simulink model "Kite_sim_actuation"  (R2022b)
settings: Solver=ode15s  StartTime=0.0  StopTime=120  FixedStep=Ts_10ms  RelTol=1e-3
InitFcn:
  | clc
  | eval('SimPrm')
StopFcn:
  | figure,plot3(Position.signals.values(:,1),Position.signals.values(:,2),Position.signals.values(:,3),'k'),grid on,hold on
  | plot3(0,0,0,'k*')
  | plot3([0, Position.signals.values(end,1)],...
  |       [0, Position.signals.values(end,2)],...
  |       [0, Position.signals.values(end,3)], 'b-o')
  | xlabel('X (m)'), ylabel('Y (m)'), zlabel('Z (m)')
  | SmoothWindPlot
values from neighbouring files (symbols this model uses):
  alpha_0 = 2.5*pi/180    (= 0.0436332312999)    [SimPrm.m]
  alpha_max = 18*pi/180    (= 0.314159265359)    [SimPrm.m]
  alpha_min = -8*pi/180    (= -0.13962634016)    [SimPrm.m]
  alpha_var = [-8.5 0 6 10 14 16 18 20]*pi/180'    [SimPrm.m]
  area = 9    [SimPrm.m]
  CD_Line = 1.2    [SimPrm.m]
  CD_var = [0.010 0.013 0.048 0.083     0.128 0.154 0.181 0.218]'    [SimPrm.m]
  CL_var = [-0.147 0.332 0.652 0.838     0.99 1.052 1.084 1.032]'*0.8    [SimPrm.m]
  ConstWindX = 5    [SimPrm.m]
  ConstWindY = 0    [SimPrm.m]
  ConstWindZ = 0    [SimPrm.m]
  g = 9.81    [SimPrm.m]
  gamma_fb_K = 2*2.8*0.01    (= 0.056)    [SimPrm.m]
  HLC2dl = -4    [SimPrm.m]
  HLC_input_max = 0.25    [SimPrm.m]
  init_stat = [60*pi/180 1*pi/180      1*pi/180 1*pi/180      50 0]    [SimPrm.m]
  K_r = 1000    [SimPrm.m]
  Line_density = 970    [SimPrm.m]
  Line_diameter = 0.003    [SimPrm.m]
  mass = 2.4    [SimPrm.m]
  n_line = 3    [SimPrm.m]
  r_ref = init_stat(5)    [SimPrm.m]
  rho = 1.2    [SimPrm.m]
  Targets_matrix = [0.3 -0.3 ... (first row only)    [SimPrm.m]
  Ts_10ms = 1e-2    (= 0.01)    [SimPrm.m]
  wingspan = 2    [SimPrm.m]
undefined symbols (not defined in the file or in its folder): WxFncH, WyFncH
settings Model: PauseTimes=60  Creator=Philip Hu  LastModifiedBy=matte
settings SolverCC: AlgebraicLoopSolver=TrustRegion  MinimalZcImpactIntegration=on
settings DataIOCC: SaveFormat=Array  SignalLoggingSaveFormat=ModelDataLogs  SaveOutput=off  SignalLogging=off  SaveTime=off  ReturnWorkspaceOutputs=off
settings OptimizationCC: BufferReuse=off  GlobalBufferReuse=off  ExpressionFolding=off  ExpressionDepthLimit=2147483647  LocalBlockOutputs=off
settings DebuggingCC: ReadBeforeWriteMsg=DisableAll  WriteAfterWriteMsg=DisableAll  WriteAfterReadMsg=DisableAll  UnderspecifiedInitializationDetection=Classic  MergeDetectMultiDrivingBlocksExec=none  SolverPrmCheckMsg=warning  MultiTaskDSMMsg=none  UnconnectedInputMsg=warning  UnconnectedOutputMsg=warning  UnconnectedLineMsg=warning  StateNameClashWarn=warning  SFUnexpectedBacktrackingDiag=warning  SFNoUnconditionalDefaultTransitionDiag=warning  SFExecutionAtInitializationDiag=none  ArithmeticOperatorsInVariantConditions=warning
settings HardwareCC: ProdBitPerPointer=32  ProdBitPerSizeT=32  ProdBitPerPtrDiffT=32  ProdLargestAtomicFloat=None  ProdWordSize=32  ProdLongLongMode=on  ProdHWDeviceType=Generic->32-bit x86 compatible
settings ModelReferenceCC: UpdateModelReferenceTargets=IfOutOfDate  EnableRefExpFcnMdlSchedulingChecks=on  PropagateSignalLabelsOutOfModel=off
settings SFSimCC: SFSimEcho=off  SimUseLocalCustomCode=off  SimParseCustomCode=off  CustomCodeUndefinedFunction=UseInterfaceOnly
settings RTWCC: Description=Simulink Real-Time  SystemTargetFile=slrt.tlc  TemplateMakefile=slrt_default_tmf  RTWUseLocalCustomCode=off  RTWCompilerOptimization=on
settings CodeAppCC: StateflowObjectComments=on
settings SimulinkRealTimeCC: OptimizeReductions=off  RL32ObjectName=HAWE  xPCisModelTimeout=off  xPCModelTimeoutSecs=20
settings ConfigComp: CovMetricSettings=dw  CovSaveCumulativeToWorkspaceVar=on  CovSaveSingleToWorkspaceVar=on  CovExternalEMLEnable=off

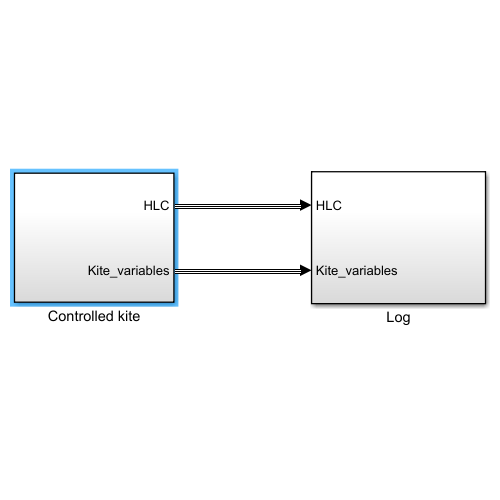
[thumbnail: Simulink's stored preview of the top-level diagram]
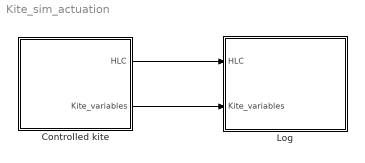
== system Kite_sim_actuation ==
  Controlled kite : Subsystem
  Log : Subsystem
  wires:
  Controlled kite/1(HLC) -> Log/1(HLC)
  Controlled kite/2(Kite_variables) -> Log/2(Kite_variables)

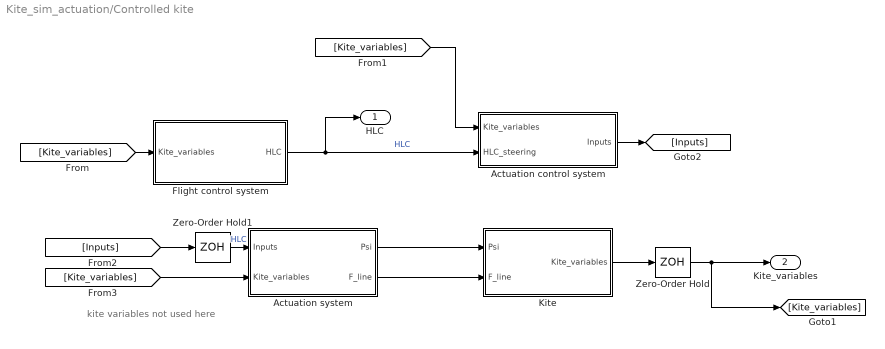
== system Kite_sim_actuation/Controlled kite ==
  note: kite variables not used here
  Actuation control system : Subsystem
  Actuation system : Subsystem
  Flight control system : Subsystem
  Kite : Subsystem
  Zero-Order Hold : ZeroOrderHold  SampleTime=Ts_10ms
  Zero-Order Hold1 : ZeroOrderHold  SampleTime=Ts_10ms
  HLC : Outport
  Kite_variables : Outport  Port=2
  wires:
  Kite/1(Kite_variables) -> Zero-Order Hold/1
  Flight control system/1(HLC) -> Actuation control system/2(HLC_steering), HLC/1  "HLC"
  Zero-Order Hold/1 -> [Kite_variables], Kite_variables/1
  [Kite_variables] -> Flight control system/1(Kite_variables)
  [Kite_variables] -> Actuation control system/1(Kite_variables)
  Actuation control system/1(Inputs) -> [Inputs]
  [Inputs] -> Zero-Order Hold1/1
  Zero-Order Hold1/1 -> Actuation system/1(Inputs)  "HLC"
  Actuation system/2(F_line) -> Kite/2(F_line)
  Actuation system/1(Psi) -> Kite/1(Psi)
  [Kite_variables] -> Actuation system/2(Kite_variables)

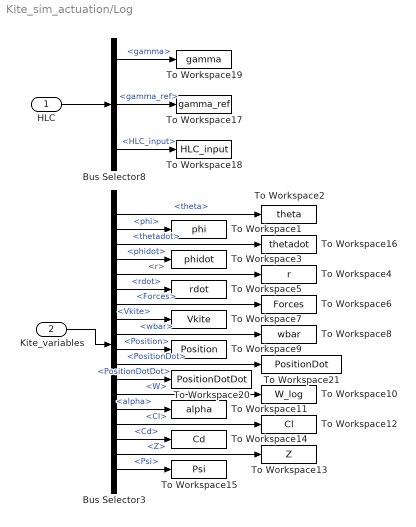
== system Kite_sim_actuation/Log ==
  HLC : Inport
  Kite_variables : Inport  Port=2
  Bus Selector3 : BusSelector  OutputSignals=states.theta,states.phi,states.thetadot,states.phidot,states.r,states.rdot,Forces,Vkite,wbar,Position,PositionDot,PositionDotDot,W,alpha,Cl,Cd,Z,Psi
  Bus Selector8 : BusSelector  OutputSignals=gamma,gamma_ref,HLC_input
  To Workspace1 : ToWorkspace  VariableName=phi  SaveFormat=Structure With Time  SampleTime=-1
  To Workspace10 : ToWorkspace  VariableName=W_log  SaveFormat=Structure With Time  SampleTime=-1
  To Workspace11 : ToWorkspace  VariableName=alpha  SaveFormat=Structure With Time  SampleTime=-1
  To Workspace12 : ToWorkspace  VariableName=Cl  SaveFormat=Structure With Time  SampleTime=-1
  To Workspace13 : ToWorkspace  VariableName=Z  SaveFormat=Structure With Time  SampleTime=-1
  To Workspace14 : ToWorkspace  VariableName=Cd  SaveFormat=Structure With Time  SampleTime=-1
  To Workspace15 : ToWorkspace  VariableName=Psi  SaveFormat=Structure With Time  SampleTime=-1
  To Workspace16 : ToWorkspace  VariableName=thetadot  SaveFormat=Structure With Time  SampleTime=-1
  To Workspace17 : ToWorkspace  VariableName=gamma_ref  SaveFormat=Structure With Time  SampleTime=-1
  To Workspace18 : ToWorkspace  VariableName=HLC_input  SaveFormat=Structure With Time  SampleTime=-1
  To Workspace19 : ToWorkspace  VariableName=gamma  SaveFormat=Structure With Time  SampleTime=-1
  To Workspace2 : ToWorkspace  VariableName=theta  SaveFormat=Structure With Time  SampleTime=-1
  To Workspace20 : ToWorkspace  VariableName=PositionDotDot  SaveFormat=Structure With Time  SampleTime=-1
  To Workspace21 : ToWorkspace  VariableName=PositionDot  SaveFormat=Structure With Time  SampleTime=-1
  To Workspace3 : ToWorkspace  VariableName=phidot  SaveFormat=Structure With Time  SampleTime=-1
  To Workspace4 : ToWorkspace  VariableName=r  SaveFormat=Structure With Time  SampleTime=-1
  To Workspace5 : ToWorkspace  VariableName=rdot  SaveFormat=Structure With Time  SampleTime=-1
  To Workspace6 : ToWorkspace  VariableName=Forces  SaveFormat=Structure With Time  SampleTime=-1
  To Workspace7 : ToWorkspace  VariableName=Vkite  SaveFormat=Structure With Time  SampleTime=-1
  To Workspace8 : ToWorkspace  VariableName=wbar  SaveFormat=Structure With Time  SampleTime=-1
  To Workspace9 : ToWorkspace  VariableName=Position  SaveFormat=Structure With Time  SampleTime=-1
  wires:
  HLC/1 -> Bus Selector8/1
  Kite_variables/1 -> Bus Selector3/1
  Bus Selector3/5 -> To Workspace4/1  "<r>"
  Bus Selector3/6 -> To Workspace5/1  "<rdot>"
  Bus Selector3/7 -> To Workspace6/1  "<Forces>"
  Bus Selector3/8 -> To Workspace7/1  "<Vkite>"
  Bus Selector3/9 -> To Workspace8/1  "<wbar>"
  Bus Selector3/10 -> To Workspace9/1  "<Position>"
  Bus Selector3/13 -> To Workspace10/1  "<W>"
  Bus Selector3/14 -> To Workspace11/1  "<alpha>"
  Bus Selector3/15 -> To Workspace12/1  "<Cl>"
  Bus Selector3/16 -> To Workspace14/1  "<Cd>"
  Bus Selector3/18 -> To Workspace15/1  "<Psi>"
  Bus Selector3/1 -> To Workspace2/1  "<theta>"
  Bus Selector3/2 -> To Workspace1/1  "<phi>"
  Bus Selector3/4 -> To Workspace3/1  "<phidot>"
  Bus Selector3/17 -> To Workspace13/1  "<Z>"
  Bus Selector3/3 -> To Workspace16/1  "<thetadot>"
  Bus Selector8/3 -> To Workspace18/1  "<HLC_input>"
  Bus Selector8/2 -> To Workspace17/1  "<gamma_ref>"
  Bus Selector8/1 -> To Workspace19/1  "<gamma>"
  Bus Selector3/12 -> To Workspace20/1  "<PositionDotDot>"
  Bus Selector3/11 -> To Workspace21/1  "<PositionDot>"

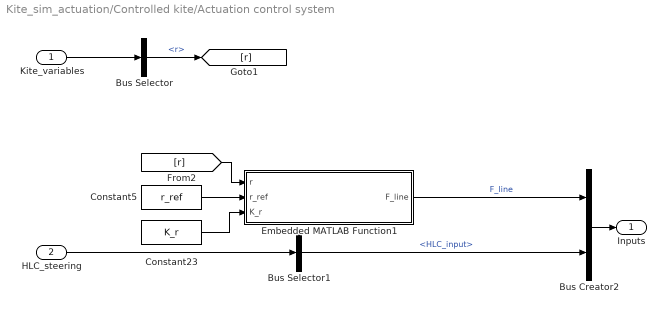
== system Kite_sim_actuation/Controlled kite/Actuation control system ==
  Kite_variables : Inport
  HLC_steering : Inport  Port=2
  Bus Creator2 : BusCreator  Inputs=2
  Bus Selector : BusSelector  OutputSignals=states.r
  Bus Selector1 : BusSelector  OutputSignals=HLC_input
  Constant23 : Constant  Value=K_r
  Constant5 : Constant  Value=r_ref
  Embedded MATLAB Function1 : MATLAB Function  TreatAsAtomicUnit=on
  Inputs : Outport
  wires:
  Embedded MATLAB Function1/1(F_line) -> Bus Creator2/1  "F_line"
  [r] -> Embedded MATLAB Function1/1(r)
  Constant5/1 -> Embedded MATLAB Function1/2(r_ref)
  Constant23/1 -> Embedded MATLAB Function1/3(K_r)
  Kite_variables/1 -> Bus Selector/1
  Bus Selector/1 -> [r]  "<r>"
  HLC_steering/1 -> Bus Selector1/1
  Bus Creator2/1 -> Inputs/1
  Bus Selector1/1 -> Bus Creator2/2  "<HLC_input>"

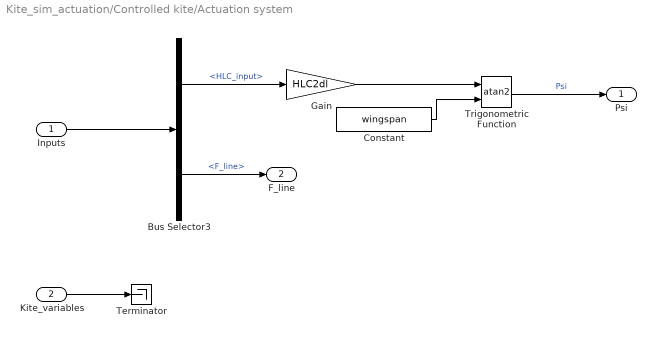
== system Kite_sim_actuation/Controlled kite/Actuation system ==
  Inputs : Inport
  Kite_variables : Inport  Port=2
  Bus Selector3 : BusSelector  OutputSignals=HLC_input,F_line
  Constant : Constant  Value=wingspan
  Gain : Gain  Gain=HLC2dl
  Terminator : Terminator
  Trigonometric Function : Trigonometry  Operator=atan2
  Psi : Outport
  F_line : Outport  Port=2
  wires:
  Bus Selector3/1 -> Gain/1  "<HLC_input>"
  Trigonometric Function/1 -> Psi/1  "Psi"
  Constant/1 -> Trigonometric Function/2
  Gain/1 -> Trigonometric Function/1
  Inputs/1 -> Bus Selector3/1
  Bus Selector3/2 -> F_line/1  "<F_line>"
  Kite_variables/1 -> Terminator/1

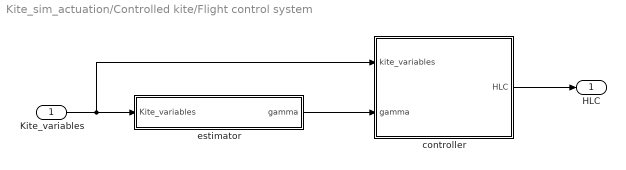
== system Kite_sim_actuation/Controlled kite/Flight control system ==
  Kite_variables : Inport
  controller : Subsystem
  estimator : Subsystem
  HLC : Outport
  wires:
  estimator/1(gamma) -> controller/2(gamma)
  controller/1(HLC) -> HLC/1
  Kite_variables/1 -> estimator/1(Kite_variables), controller/1(kite_variables)

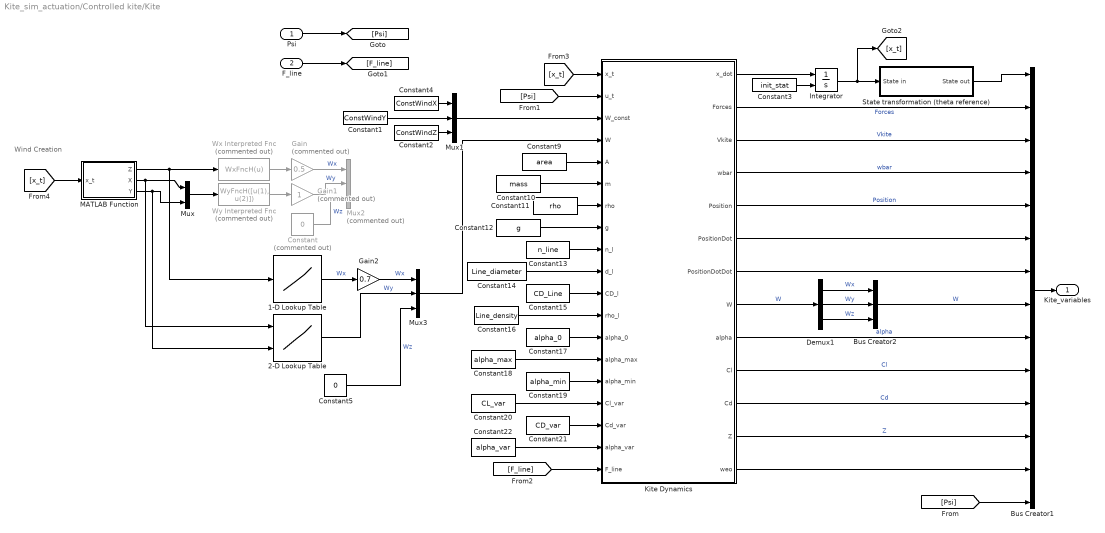
== system Kite_sim_actuation/Controlled kite/Kite ==
  note: Wind Creation
  Psi : Inport
  F_line : Inport  Port=2
  1-D Lookup Table : Lookup_n-D  NumberOfTableDimensions=1  BreakpointsForDimension1=[0;5;10;15;20;25;40;50]  Table=[0 2 8 10 12 20 20 20]  InterpMethod=Cubic spline  ExtrapMethod=Cubic spline  InternalRulePriority=Speed  RndMeth=Simplest
  2-D Lookup Table : Lookup_n-D  BreakpointsForDimension1=[0 25 30 50 60 80 100]  BreakpointsForDimension2=[-50;-20;-10;0;10;20;50]  Table=[0 0 0 0 0 0 0;0 0 0 0 0 0 0;0 0 5 0 0 0 0;0 0 0 0 10 0 0;0 0 0 0 0 0 0;0 -10 0 0 0 0 0;0 0 0 0 0 0 0]  InterpMethod=Cubic spline  ExtrapMethod=Cubic spline  InternalRulePriority=Speed  RndMeth=Simplest
      settings: InputPortMap=u0,u1
  Bus Creator1 : BusCreator  Inputs=14
  Bus Creator2 : BusCreator  Inputs=3
  Constant : Constant  Commented=on  Value=0
  Constant1 : Constant  Value=ConstWindY
  Constant10 : Constant  Value=mass
  Constant11 : Constant  Value=rho
  Constant12 : Constant  Value=g
  Constant13 : Constant  Value=n_line
  Constant14 : Constant  Value=Line_diameter
  Constant15 : Constant  Value=CD_Line
  Constant16 : Constant  Value=Line_density
  Constant17 : Constant  Value=alpha_0
  Constant18 : Constant  Value=alpha_max
  Constant19 : Constant  Value=alpha_min
  Constant2 : Constant  Value=ConstWindZ
  Constant20 : Constant  Value=CL_var
  Constant21 : Constant  Value=CD_var
  Constant22 : Constant  Value=alpha_var
  Constant3 : Constant  Value=init_stat
  Constant4 : Constant  Value=ConstWindX
  Constant5 : Constant  Value=0
  Constant9 : Constant  Value=area
  Demux1 : Demux  Outputs=3
  Gain : Gain  Commented=on  Gain=0.5
  Gain1 : Gain  Commented=on
  Gain2 : Gain  Gain=0.7
  Integrator : Integrator  InitialConditionSource=external
  Kite Dynamics : MATLAB Function  TreatAsAtomicUnit=on
  MATLAB Function : MATLAB Function  TreatAsAtomicUnit=on
  Mux : Mux  Inputs=2
  Mux1 : Mux  Inputs=3
  Mux2 : Mux  Commented=on  Inputs=3
  Mux3 : Mux  Inputs=3
  State transformation (theta reference) : Subsystem
  Wx Interpreted Fnc : MATLABFcn  Commented=on  MATLABFcn=WxFncH(u)  OutputDimensions=1  OutputSignalType=real  Output1D=off
  Wy Interpreted Fnc : MATLABFcn  Commented=on  MATLABFcn=WyFncH([u(1), u(2)])  OutputDimensions=1  OutputSignalType=real  Output1D=off
  Kite_variables : Outport
  wires:
  State transformation (theta reference)/1(State out) -> Bus Creator1/1
  Constant2/1 -> Mux1/3
  Constant1/1 -> Mux1/2
  Constant4/1 -> Mux1/1
  Mux1/1 -> Kite Dynamics/3(W_const)
  Constant9/1 -> Kite Dynamics/5(A)
  Constant10/1 -> Kite Dynamics/6(m)
  Constant11/1 -> Kite Dynamics/7(rho)
  Constant12/1 -> Kite Dynamics/8(g)
  Constant13/1 -> Kite Dynamics/9(n_l)
  Constant14/1 -> Kite Dynamics/10(d_l)
  Constant15/1 -> Kite Dynamics/11(CD_l)
  Constant16/1 -> Kite Dynamics/12(rho_l)
  Constant18/1 -> Kite Dynamics/14(alpha_max)
  Constant20/1 -> Kite Dynamics/16(Cl_var)
  Constant22/1 -> Kite Dynamics/18(alpha_var)
  Constant17/1 -> Kite Dynamics/13(alpha_0)
  Constant19/1 -> Kite Dynamics/15(alpha_min)
  Constant21/1 -> Kite Dynamics/17(Cd_var)
  [F_line] -> Kite Dynamics/19(F_line)
  Bus Creator1/1 -> Kite_variables/1
  Kite Dynamics/2(Forces) -> Bus Creator1/2  "Forces"
  Kite Dynamics/3(Vkite) -> Bus Creator1/3  "Vkite"
  Kite Dynamics/4(wbar) -> Bus Creator1/4  "wbar"
  Kite Dynamics/5(Position) -> Bus Creator1/5  "Position"
  Kite Dynamics/8(W) -> Demux1/1  "W"
  Kite Dynamics/9(alpha) -> Bus Creator1/9  "alpha"
  Kite Dynamics/10(Cl) -> Bus Creator1/10  "Cl"
  Kite Dynamics/11(Cd) -> Bus Creator1/11  "Cd"
  Kite Dynamics/12(Z) -> Bus Creator1/12  "Z"
  Integrator/1 -> [x_t], State transformation (theta reference)/1(State in)
  Constant3/1 -> Integrator/2
  Kite Dynamics/1(x_dot) -> Integrator/1
  Kite Dynamics/13(weo) -> Bus Creator1/13
  Demux1/1 -> Bus Creator2/1  "Wx"
  Demux1/2 -> Bus Creator2/2  "Wy"
  Demux1/3 -> Bus Creator2/3  "Wz"
  Bus Creator2/1 -> Bus Creator1/8  "W"
  [Psi] -> Bus Creator1/14
  [Psi] -> Kite Dynamics/2(u_t)
  Psi/1 -> [Psi]
  F_line/1 -> [F_line]
  Constant/1 -> Mux2/3  "Wz"
  MATLAB Function/1(Z) -> 1-D Lookup Table/1, Wx Interpreted Fnc/1
  Mux/1 -> Wy Interpreted Fnc/1
  MATLAB Function/2(X) -> 2-D Lookup Table/1, Mux/1
  MATLAB Function/3(Y) -> 2-D Lookup Table/2, Mux/2
  Wx Interpreted Fnc/1 -> Gain/1
  Gain/1 -> Mux2/1  "Wx"
  Wy Interpreted Fnc/1 -> Gain1/1
  Gain1/1 -> Mux2/2  "Wy"
  [x_t] -> Kite Dynamics/1(x_t)
  [x_t] -> MATLAB Function/1(x_t)
  2-D Lookup Table/1 -> Mux3/2  "Wy"
  1-D Lookup Table/1 -> Gain2/1  "Wx"
  Constant5/1 -> Mux3/3  "Wz"
  Mux3/1 -> Kite Dynamics/4("W ")
  Gain2/1 -> Mux3/1  "Wx"
  Kite Dynamics/7(PositionDotDot) -> Bus Creator1/7
  Kite Dynamics/6(PositionDot) -> Bus Creator1/6

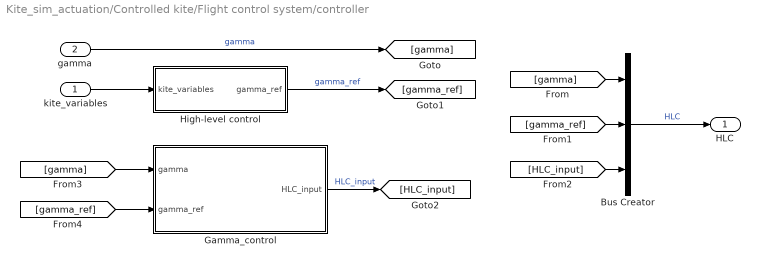
== system Kite_sim_actuation/Controlled kite/Flight control system/controller ==
  kite_variables : Inport
  gamma : Inport  Port=2
  Bus Creator : BusCreator  Inputs=3
  Gamma_control : Subsystem
  High-level control : Subsystem
  HLC : Outport
  wires:
  Bus Creator/1 -> HLC/1  "HLC"
  High-level control/1(gamma_ref) -> [gamma_ref]  "gamma_ref"
  kite_variables/1 -> High-level control/1(kite_variables)
  gamma/1 -> [gamma]  "gamma"
  [gamma] -> Bus Creator/1
  Gamma_control/1(HLC_input) -> [HLC_input]  "HLC_input"
  [gamma_ref] -> Bus Creator/2
  [HLC_input] -> Bus Creator/3
  [gamma] -> Gamma_control/1(gamma)
  [gamma_ref] -> Gamma_control/2(gamma_ref)

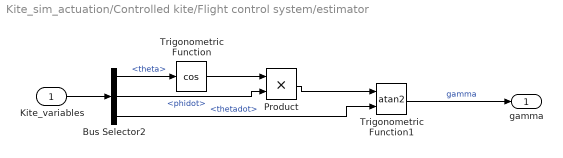
== system Kite_sim_actuation/Controlled kite/Flight control system/estimator ==
  Kite_variables : Inport
  Bus Selector2 : BusSelector  OutputSignals=states.theta,states.phidot,states.thetadot
  Product : Product  RndMeth=Zero
  Trigonometric Function : Trigonometry  Operator=cos
  Trigonometric Function1 : Trigonometry  Operator=atan2
  gamma : Outport
  wires:
  Kite_variables/1 -> Bus Selector2/1
  Bus Selector2/3 -> Trigonometric Function1/2  "<thetadot>"
  Bus Selector2/1 -> Trigonometric Function/1  "<theta>"
  Bus Selector2/2 -> Product/2  "<phidot>"
  Product/1 -> Trigonometric Function1/1
  Trigonometric Function1/1 -> gamma/1  "gamma"
  Trigonometric Function/1 -> Product/1

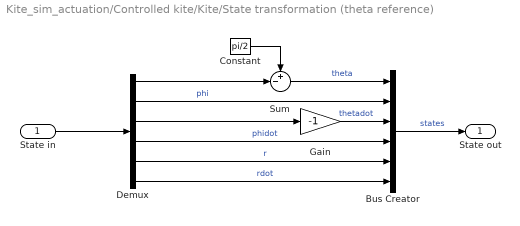
== system Kite_sim_actuation/Controlled kite/Kite/State transformation (theta reference) ==
  State in : Inport
  Bus Creator : BusCreator  Inputs=6
  Constant : Constant  Value=pi/2
  Demux : Demux  Outputs=6
  Gain : Gain  Gain=-1
  Sum : Sum  Inputs=+-|
  State out : Outport
  wires:
  Demux/2 -> Bus Creator/2  "phi"
  Demux/3 -> Gain/1
  Demux/4 -> Bus Creator/4  "phidot"
  Demux/5 -> Bus Creator/5  "r"
  Demux/6 -> Bus Creator/6  "rdot"
  Constant/1 -> Sum/1
  Demux/1 -> Sum/2
  Sum/1 -> Bus Creator/1  "theta"
  Gain/1 -> Bus Creator/3  "thetadot"
  State in/1 -> Demux/1
  Bus Creator/1 -> State out/1  "states"

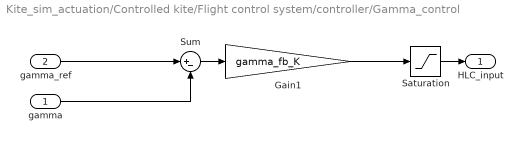
== system Kite_sim_actuation/Controlled kite/Flight control system/controller/Gamma_control ==
  gamma : Inport
  gamma_ref : Inport  Port=2
  Gain1 : Gain  Gain=gamma_fb_K
  Saturation : Saturate  UpperLimit=HLC_input_max  LowerLimit=-HLC_input_max
  Sum : Sum  Inputs=|+-
  HLC_input : Outport
  wires:
  Sum/1 -> Gain1/1
  Gain1/1 -> Saturation/1
  gamma_ref/1 -> Sum/1
  Saturation/1 -> HLC_input/1
  gamma/1 -> Sum/2

== system Kite_sim_actuation/Controlled kite/Flight control system/controller/High-level control ==
  kite_variables : Inport
  Bus Selector3 : BusSelector  OutputSignals=states.theta,states.phi
  Guidance : Subsystem
  gamma_ref : Outport
  wires:
  kite_variables/1 -> Bus Selector3/1
  Bus Selector3/1 -> Guidance/1(theta)  "<theta>"
  Bus Selector3/2 -> Guidance/2(phi)  "<phi>"
  Guidance/1(gamma_ref) -> gamma_ref/1  "gamma_ref"

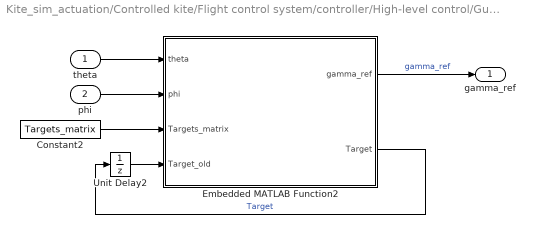
== system Kite_sim_actuation/Controlled kite/Flight control system/controller/High-level control/Guidance ==
  theta : Inport
  phi : Inport  Port=2
  Constant2 : Constant  Value=Targets_matrix
  Embedded MATLAB Function2 : MATLAB Function  TreatAsAtomicUnit=on
  Unit Delay2 : UnitDelay  InitialCondition=1  SampleTime=-1  HasFrameUpgradeWarning=on
  gamma_ref : Outport
  wires:
  Embedded MATLAB Function2/1(gamma_ref) -> gamma_ref/1  "gamma_ref"
  Embedded MATLAB Function2/2(Target) -> Unit Delay2/1  "Target"
  theta/1 -> Embedded MATLAB Function2/1(theta)
  phi/1 -> Embedded MATLAB Function2/2(phi)
  Constant2/1 -> Embedded MATLAB Function2/3(Targets_matrix)
  Unit Delay2/1 -> Embedded MATLAB Function2/4(Target_old)

== matlab function Kite_sim_actuation/Controlled kite/Flight control system/controller/High-level control/Guidance/Embedded MATLAB Function2 ==
  data: theta input; phi input; Targets_matrix input; gamma_ref output; Target output; Target_old input
function [gamma_ref,Target]=kite_guidance(theta,...
                                         phi,...
                                         Targets_matrix,...
                                         Target_old)%#eml

% Gamma reference computation strategy (based on theta, phi and Target; 
% theta and phi of the targets to be included in Targets_matrix, 
% e.g. the i-th row has theta and phi of the 
% i-th target; theta_min is for emergency situation)

if phi > Targets_matrix(2,2) % Regular switch, over pos limit
    Target = 1;
elseif phi < Targets_matrix(1,2) % Regular switch, below neg limit
    Target = 2;
else
    Target = Target_old;
end

% Calculate gamma_ref
theta_t = Targets_matrix(Target,1);
phi_t   = Targets_matrix(Target,2);
gamma_ref = atan2((phi_t - phi)*cos(theta),theta_t - theta);

== matlab function Kite_sim_actuation/Controlled kite/Actuation control system/Embedded MATLAB Function1 ==
  data: r input; F_line output; r_ref input; K_r input
function F_line=...
    line_ctrl(r,r_ref,K_r)%#eml


F_line=[0;0;-K_r*(r_ref-r)];
F_line(3,1)=max(0,F_line(3,1)); % cable traction force (always positive and subtracted to other forces)

== matlab function Kite_sim_actuation/Controlled kite/Kite/MATLAB Function ==
  data: Z output; x_t input; X output; Y output
function [Z, X, Y] = KitePosition(x_t)

theta       =       x_t(1);
phi         =       x_t(2);
r           =       x_t(5);


X = r*sin(theta)*cos(phi);
Y = r*sin(theta)*sin(phi);
Z = max(1,r*cos(theta));

== matlab function Kite_sim_actuation/Controlled kite/Kite/Kite Dynamics ==
  data: x_t input; x_dot output; u_t input; W_const input; W input; Forces output; A input; m input; rho input; g input; n_l input; d_l input; CD_l input; rho_l input; alpha_0 input; alpha_max input; alpha_min input; Cl_var input; Cd_var input; alpha_var input; F_line input; Vkite output; wbar output; Position output; PositionDot output; PositionDotDot output; W output; alpha output; Cl output; Cd output; Z output; weo output
function [x_dot,Forces,Vkite,wbar,Position,PositionDot, PositionDotDot,W,alpha,Cl,Cd,Z,weo]=...
    kite_dynamics(x_t,u_t,W_const,W,A,m,rho,g,n_l,...
    d_l,CD_l,rho_l,alpha_0,alpha_max,alpha_min,Cl_var,Cd_var,alpha_var,F_line)%#eml

% Discrete-time kite dynamics with fixed KSU (e.g. for
% KE-yoyo configuration)
%
% Author: L. Fagiano
% August 1 2012

theta       =       x_t(1);
phi         =       x_t(2);
r           =       x_t(5);
thetadot    =       x_t(3);
phidot      =       x_t(4);
rdot        =       x_t(6);
psi         =       u_t;

Z=max(1,r*cos(theta));

%W = W + W_const;
                                                                                                                      
ep=[...
    cos(theta)*cos(phi)  -sin(phi)    sin(theta)*cos(phi)
    cos(theta)*sin(phi)  cos(phi)     sin(theta)*sin(phi)
    -sin(theta)          0            cos(theta)
    ];                               % local coordinate system -> nominal wind coordinate system


Position=r*ep(:,3);                   % position of kite

wp=ep'*W;                           % wind in local coordinate system

vp=[...
    r*thetadot
    r*sin(theta)*phidot
    rdot
    ];                                % apparent wind due to kite movement (local system)
vp=-vp;

wep=vp+wp;                          % calculate effective wind we (in local coordinates)

weo=ep*wep;                         % effective wind we in nominal wind coordinate system
weobar=norm(weo);                   % norm of effective wind speed

epp=zeros(3,3);

epp(:,1)=wep;                       % epp(:,1) pointing in projected direction of effective wind wep
epp(3,1)=0;
wbar=norm(epp(:,1));
wbar=max(1e-8,wbar);                % saturation on minimal wind tangential to the sphere

epp(:,1)=epp(:,1)/wbar;             % projected coordinate system - axis 1

epp(:,3)=[0;0;1];                   % projected coordinate system - axis 3

epp(:,2)=[-epp(2,1),epp(1,1),0];    % projected coordinate system - axis 2

wepp=epp'*wep;                      % translate wep in new system

ratio=wepp(3)*tan(psi)/wepp(1);

ratio=min(1,ratio);                 % saturation on sine of eta angle
ratio=max(-1,ratio);                % saturation on sine of eta angle

eta = asin(ratio);

etpp=[cos(psi)*(-sin(eta));cos(psi)*(cos(eta));sin(psi)];

edpp=wepp/norm(wepp);               % drag direction
ldpp=outprod(edpp,etpp);            % lift direction

edp=epp*edpp;                       % Turn edpp into local system
ldp=epp*ldpp;                       % Turn ldpp into local system

Pdyn=weobar*weobar*1/2*rho;

tan_d_alpha=wepp(3,1)/wepp(1,1);
d_alpha=atan(tan_d_alpha);          % angle of attack variation

alpha=alpha_0+d_alpha;              % angle of attack
alpha=min(alpha_max,alpha);         % angle of attack saturation
alpha=max(alpha_min,alpha);         % angle of attack saturation

Cl=interp1(alpha_var,Cl_var,alpha,'linear','extrap'); % lift coefficient
Cd=interp1(alpha_var,Cd_var,alpha,'linear','extrap'); % drag coefficient


Fl=Pdyn*A*Cl*ldp;                   % lift force

Drag_line=Pdyn*1/4*cos(d_alpha)*r*d_l*n_l*CD_l;     % Cable drag force
Fd_tot=(Pdyn*A*Cd+Drag_line)*edp;                   % Total drag force

Fapp=m*[phidot^2*r*sin(theta)*cos(theta)-2*rdot*thetadot;
    -2*rdot*phidot*sin(theta) - 2*thetadot*phidot*r*cos(theta);
    r*thetadot^2+r*phidot^2*sin(theta)^2]; % apparent forces

Fgrav=(m+n_l*rho_l*pi*r*d_l^2/4)*g*[sin(theta);0;-cos(theta)]; % gravity forces

% F_cavo=[0;0;(Fl(3,1)+Fapp(3,1)+Fd_tot(3,1)+Fgrav(3,1))-K_r*(r_slope-rdot)];
% F_cavo(3,1)=max(0,F_cavo(3,1)); % cable traction force (always positive and subtracted to other forces)

F_tot=Fl+Fd_tot+Fapp+Fgrav-F_line;

thetadotdot = F_tot(1,1)/(m*r);
phidotdot = F_tot(2,1)/(m*r*sin(theta));
rdotdot = F_tot(3,1)/m;

x_dot=[ thetadot;                           % theta dot
        phidot;                             % phi dot
        thetadotdot;                        % theta dotdot
        phidotdot;                          % phi dotdot
        rdot;                               % r dot
        rdotdot];                           % r dotdot

PositionDot = rdComputation(r, theta, phi, rdot, thetadot, phidot);
PositionDotDot = rddComputation(r, theta, phi, rdot, thetadot, phidot, rdotdot, thetadotdot, phidotdot);

Fl_nom = ep*Fl;                             % Moving Fl back to nominal ref sys
Fd_tot_nom = ep*Fd_tot;                     % Moving Fd back to nominal ref sys

Forces=[F_tot;Fl_nom;Fd_tot_nom;F_line(3,1)];
Vkite=norm(vp);

function c=outprod(a, b)
c=double(zeros(3,1));
c(1)=  a(2)*b(3) - a(3)*b(2);
c(2)=  a(3)*b(1) - a(1)*b(3);
c(3)=  a(1)*b(2) - a(2)*b(1);
c=c(:);

function rdotdot = rddComputation(L, th, ph, L_dot, th_dot, ph_dot, L_dotdot, th_dotdot, ph_dotdot)
rdotdot = [cos(ph)*sin(th)*L_dotdot - sin(ph)*sin(th)*L*ph_dotdot + 2*cos(ph)*cos(th)*th_dot*L_dot - 2*sin(ph)*sin(th)*ph_dot*L_dot - cos(ph)*sin(th)*L*(ph_dot)^2 - cos(ph)*sin(th)*L*(th_dot)^2 + cos(ph)*cos(th)*L*th_dotdot - 2*cos(th)*sin(ph)*L*th_dot*ph_dot;...
           sin(ph)*sin(th)*L_dotdot + 2*cos(ph)*sin(th)*ph_dot*L_dot + 2*cos(th)*sin(ph)*th_dot*L_dot - sin(ph)*sin(th)*L*(ph_dot)^2 - sin(ph)*sin(th)*L*(th_dot)^2 + cos(ph)*sin(th)*L*ph_dotdot + cos(th)*sin(ph)*L*th_dotdot + 2*cos(ph)*cos(th)*L*th_dot*ph_dot;...
           cos(th)*L_dotdot - 2*sin(th)*th_dot*L_dot - cos(th)*L*(th_dot)^2 - sin(th)*L*th_dotdot];

function rdot = rdComputation(L, th, ph, L_dot, th_dot, ph_dot)
rdot = [L_dot*sin(th)*cos(ph)+L.*(th_dot.*cos(th).*cos(ph)-ph_dot.*sin(th).*sin(ph)); ... 
        L_dot.*sin(th).*sin(ph)+L.*(th_dot.*cos(th).*sin(ph)+ph_dot.*sin(th).*cos(ph)); ...
        L_dot.*cos(th)-L.*th_dot.*sin(th)];
